simulink model "cruise_control_aberta"  (R2019b)
settings: Solver=FixedStepAuto  StartTime=0.0  StopTime=100  FixedStep=1e-3  RelTol=1e-3
values from neighbouring files (symbols this model uses):
  b = f/vf    [identificarCruiseControl.m]
  m = tau*b    [identificarCruiseControl.m]
undefined symbols (not defined in the file or in its folder): d
settings Model: Creator=mmaximo  LastModifiedBy=rodri

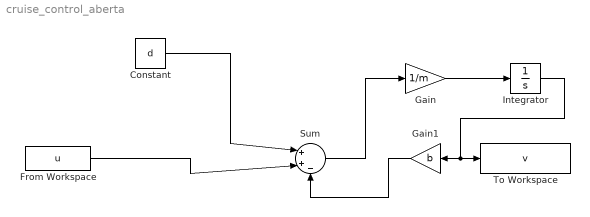
== system cruise_control_aberta ==
  Constant : Constant  Value=d
  From Workspace : FromWorkspace  VariableName=u  SampleTime=0
  Gain : Gain  Gain=1/m
  Gain1 : Gain  Gain=b
  Integrator : Integrator
  Sum : Sum  Inputs=|++-
  To Workspace : ToWorkspace  VariableName=v  SaveFormat=Structure With Time  SampleTime=-1
  wires:
  From Workspace/1 -> Sum/2
  Constant/1 -> Sum/1
  Sum/1 -> Gain/1
  Gain/1 -> Integrator/1
  Integrator/1 -> To Workspace/1, Gain1/1
  Gain1/1 -> Sum/3
